simulink model "rezervor"  (R2022b)
settings: Solver=VariableStepAuto  StartTime=0.0  StopTime=10.0  RelTol=1e-3
settings Model: Creator=fabian  LastModifiedBy=fabian

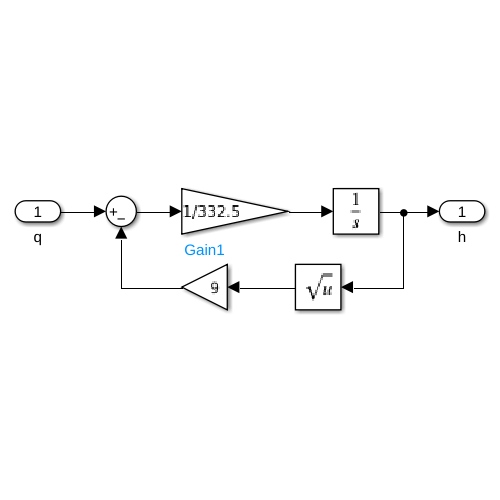
[thumbnail: Simulink's stored preview of the top-level diagram]
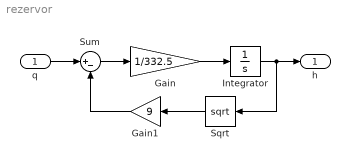
== system rezervor ==
  q : Inport
  Gain : Gain  Gain=1/332.5
  Gain1 : Gain  Gain=9
  Integrator : Integrator
  Sqrt : Sqrt
  Sum : Sum  Inputs=|+-
  h : Outport
  wires:
  q/1 -> Sum/1
  Sum/1 -> Gain/1
  Gain/1 -> Integrator/1
  Integrator/1 -> Sqrt/1, h/1
  Sqrt/1 -> Gain1/1
  Gain1/1 -> Sum/2
